simulink model "recycle1"  (R2024a)
settings: Solver=VariableStepAuto  StartTime=0.0  StopTime=100  MaxStep=0.1  RelTol=1e-3
libraries: simulink x20
(part 2 of 2)

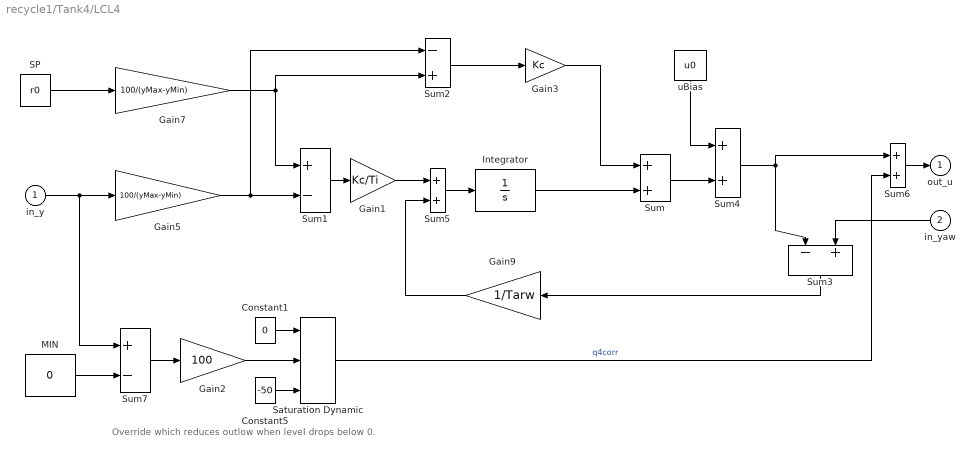
== system recycle1/Tank4/LCL4 ==
  note: Override which reduces outlow when level drops below 0.
  in_y : Inport
  in_yaw : Inport  Port=2
  Constant1 : Constant  Value=0
  Constant5 : Constant  Value=-50
  Gain1 : Gain  Gain=Kc/Ti  SaturateOnIntegerOverflow=on  OutDataTypeStr=Inherit: Same as input  ParamDataTypeStr=Inherit: Same as input
  Gain2 : Gain  Gain=100  SaturateOnIntegerOverflow=on  OutDataTypeStr=Inherit: Same as input  ParamDataTypeStr=Inherit: Same as input
  Gain3 : Gain  Gain=Kc  SaturateOnIntegerOverflow=on  OutDataTypeStr=Inherit: Same as input  ParamDataTypeStr=Inherit: Same as input
  Gain5 : Gain  Gain=100/(yMax-yMin)  SaturateOnIntegerOverflow=on  OutDataTypeStr=Inherit: Same as input  ParamDataTypeStr=Inherit: Same as input
  Gain7 : Gain  Gain=100/(yMax-yMin)  SaturateOnIntegerOverflow=on  OutDataTypeStr=Inherit: Same as input  ParamDataTypeStr=Inherit: Same as input
  Gain9 : Gain  Gain=1/Tarw  SaturateOnIntegerOverflow=on  OutDataTypeStr=Inherit: Same as input  ParamDataTypeStr=Inherit: Same as input
  Integrator : Integrator
  MIN : Constant  Value=0
  SP : Constant  Value=r0
  Saturation Dynamic : simulink/Discontinuities/Saturation Dynamic  OutMin=[]  OutMax=[]  OutDataTypeStr=Inherit: Same as second input  OutDataType=fixdt(1, 16)  OutScaling=2^-10  DoSatur=off
  Sum{,4..6} (4 alike) : Sum  InputSameDT=on  SaturateOnIntegerOverflow=on  OutDataTypeStr=Inherit: Same as first input
  Sum1 : Sum  Inputs=+-  InputSameDT=on  SaturateOnIntegerOverflow=on  OutDataTypeStr=Inherit: Same as first input
  Sum2 : Sum  Inputs=-+  InputSameDT=on  SaturateOnIntegerOverflow=on  OutDataTypeStr=Inherit: Same as first input
  Sum3 : Sum  Inputs=-+  InputSameDT=on  SaturateOnIntegerOverflow=on  OutDataTypeStr=Inherit: Same as first input
  Sum7 : Sum  Inputs=+-  InputSameDT=on  SaturateOnIntegerOverflow=on  OutDataTypeStr=Inherit: Same as first input
  uBias : Constant  Value=u0
  out_u : Outport  VectorParamsAs1DForOutWhenUnconnected=off
  wires:
  Gain3/1 -> Sum/1
  Sum5/1 -> Integrator/1
  Gain9/1 -> Sum5/2
  Gain1/1 -> Sum5/1
  Sum3/1 -> Gain9/1
  Sum/1 -> Sum4/2
  Gain5/1 -> Sum2/1, Sum1/2
  Sum2/1 -> Gain3/1
  Gain7/1 -> Sum2/2, Sum1/1
  Sum1/1 -> Gain1/1
  in_y/1 -> Sum7/1, Gain5/1
  SP/1 -> Gain7/1
  Integrator/1 -> Sum/2
  uBias/1 -> Sum4/1
  in_yaw/1 -> Sum3/2
  Constant5/1 -> Saturation Dynamic/3
  Saturation Dynamic/1 -> Sum6/2  "q4corr"
  MIN/1 -> Sum7/2
  Gain2/1 -> Saturation Dynamic/2
  Sum7/1 -> Gain2/1
  Constant1/1 -> Saturation Dynamic/1
  Sum4/1 -> Sum3/1, Sum6/1
  Sum6/1 -> out_u/1

== system recycle1/Tank5/LCH5 ==
  note: Override which reduces inflow when level excceds 100.
  in_y : Inport
  in_yaw : Inport  Port=2
  Constant1 : Constant  Value=0
  Constant5 : Constant  Value=-50
  Gain1 : Gain  Gain=Kc/Ti  SaturateOnIntegerOverflow=on  OutDataTypeStr=Inherit: Same as input  ParamDataTypeStr=Inherit: Same as input
  Gain2 : Gain  Gain=-100  SaturateOnIntegerOverflow=on  OutDataTypeStr=Inherit: Same as input  ParamDataTypeStr=Inherit: Same as input
  Gain3 : Gain  Gain=Kc  SaturateOnIntegerOverflow=on  OutDataTypeStr=Inherit: Same as input  ParamDataTypeStr=Inherit: Same as input
  Gain5 : Gain  Gain=100/(yMax-yMin)  SaturateOnIntegerOverflow=on  OutDataTypeStr=Inherit: Same as input  ParamDataTypeStr=Inherit: Same as input
  Gain7 : Gain  Gain=100/(yMax-yMin)  SaturateOnIntegerOverflow=on  OutDataTypeStr=Inherit: Same as input  ParamDataTypeStr=Inherit: Same as input
  Gain9 : Gain  Gain=1/Tarw  SaturateOnIntegerOverflow=on  OutDataTypeStr=Inherit: Same as input  ParamDataTypeStr=Inherit: Same as input
  Integrator : Integrator
  MAX : Constant  Value=100
  SP : Constant  Value=r0
  Saturation Dynamic : simulink/Discontinuities/Saturation Dynamic  OutMin=[]  OutMax=[]  OutDataTypeStr=Inherit: Same as second input  OutDataType=fixdt(1, 16)  OutScaling=2^-10  DoSatur=off
  Sum{,4..6} (4 alike) : Sum  InputSameDT=on  SaturateOnIntegerOverflow=on  OutDataTypeStr=Inherit: Same as first input
  Sum1 : Sum  Inputs=+-  InputSameDT=on  SaturateOnIntegerOverflow=on  OutDataTypeStr=Inherit: Same as first input
  Sum2 : Sum  Inputs=-+  InputSameDT=on  SaturateOnIntegerOverflow=on  OutDataTypeStr=Inherit: Same as first input
  Sum3 : Sum  Inputs=-+  InputSameDT=on  SaturateOnIntegerOverflow=on  OutDataTypeStr=Inherit: Same as first input
  Sum7 : Sum  Inputs=+-  InputSameDT=on  SaturateOnIntegerOverflow=on  OutDataTypeStr=Inherit: Same as first input
  uBias : Constant  Value=u0
  out_u : Outport  VectorParamsAs1DForOutWhenUnconnected=off
  wires:
  Gain3/1 -> Sum/1
  Sum5/1 -> Integrator/1
  Gain9/1 -> Sum5/2
  Gain1/1 -> Sum5/1
  Sum3/1 -> Gain9/1
  Sum/1 -> Sum4/2
  Sum4/1 -> Sum6/1, Sum3/1
  Gain5/1 -> Sum2/1, Sum1/2
  Sum2/1 -> Gain3/1
  Gain7/1 -> Sum2/2, Sum1/1
  Sum1/1 -> Gain1/1
  in_y/1 -> Sum7/1, Gain5/1
  SP/1 -> Gain7/1
  Integrator/1 -> Sum/2
  uBias/1 -> Sum4/1
  in_yaw/1 -> Sum3/2
  Gain2/1 -> Saturation Dynamic/2
  Constant1/1 -> Saturation Dynamic/1
  Constant5/1 -> Saturation Dynamic/3
  Sum6/1 -> out_u/1
  Saturation Dynamic/1 -> Sum6/2  "qcorr"
  Sum7/1 -> Gain2/1
  MAX/1 -> Sum7/2

== system recycle1/Tank5/LCL5 ==
  note: Override which reduces outlow when level drops below 0.
  in_y : Inport
  in_yaw : Inport  Port=2
  Constant1 : Constant  Value=0
  Constant5 : Constant  Value=-50
  Gain1 : Gain  Gain=Kc/Ti  SaturateOnIntegerOverflow=on  OutDataTypeStr=Inherit: Same as input  ParamDataTypeStr=Inherit: Same as input
  Gain2 : Gain  Gain=100  SaturateOnIntegerOverflow=on  OutDataTypeStr=Inherit: Same as input  ParamDataTypeStr=Inherit: Same as input
  Gain3 : Gain  Gain=Kc  SaturateOnIntegerOverflow=on  OutDataTypeStr=Inherit: Same as input  ParamDataTypeStr=Inherit: Same as input
  Gain5 : Gain  Gain=100/(yMax-yMin)  SaturateOnIntegerOverflow=on  OutDataTypeStr=Inherit: Same as input  ParamDataTypeStr=Inherit: Same as input
  Gain7 : Gain  Gain=100/(yMax-yMin)  SaturateOnIntegerOverflow=on  OutDataTypeStr=Inherit: Same as input  ParamDataTypeStr=Inherit: Same as input
  Gain9 : Gain  Gain=1/Tarw  SaturateOnIntegerOverflow=on  OutDataTypeStr=Inherit: Same as input  ParamDataTypeStr=Inherit: Same as input
  Integrator : Integrator
  MIN : Constant  Value=0
  SP : Constant  Value=r0
  Saturation Dynamic : simulink/Discontinuities/Saturation Dynamic  OutMin=[]  OutMax=[]  OutDataTypeStr=Inherit: Same as second input  OutDataType=fixdt(1, 16)  OutScaling=2^-10  DoSatur=off
  Sum{,4..6} (4 alike) : Sum  InputSameDT=on  SaturateOnIntegerOverflow=on  OutDataTypeStr=Inherit: Same as first input
  Sum1 : Sum  Inputs=+-  InputSameDT=on  SaturateOnIntegerOverflow=on  OutDataTypeStr=Inherit: Same as first input
  Sum2 : Sum  Inputs=-+  InputSameDT=on  SaturateOnIntegerOverflow=on  OutDataTypeStr=Inherit: Same as first input
  Sum3 : Sum  Inputs=-+  InputSameDT=on  SaturateOnIntegerOverflow=on  OutDataTypeStr=Inherit: Same as first input
  Sum7 : Sum  Inputs=+-  InputSameDT=on  SaturateOnIntegerOverflow=on  OutDataTypeStr=Inherit: Same as first input
  uBias : Constant  Value=u0
  out_u : Outport  VectorParamsAs1DForOutWhenUnconnected=off
  wires:
  Gain3/1 -> Sum/1
  Sum5/1 -> Integrator/1
  Gain9/1 -> Sum5/2
  Gain1/1 -> Sum5/1
  Sum3/1 -> Gain9/1
  Sum/1 -> Sum4/2
  Gain5/1 -> Sum2/1, Sum1/2
  Sum2/1 -> Gain3/1
  Gain7/1 -> Sum2/2, Sum1/1
  Sum1/1 -> Gain1/1
  in_y/1 -> Sum7/1, Gain5/1
  SP/1 -> Gain7/1
  Integrator/1 -> Sum/2
  uBias/1 -> Sum4/1
  in_yaw/1 -> Sum3/2
  Constant5/1 -> Saturation Dynamic/3
  Saturation Dynamic/1 -> Sum6/2  "q4corr"
  MIN/1 -> Sum7/2
  Gain2/1 -> Saturation Dynamic/2
  Sum7/1 -> Gain2/1
  Constant1/1 -> Saturation Dynamic/1
  Sum4/1 -> Sum3/1, Sum6/1
  Sum6/1 -> out_u/1
